simulink model "M2C_IM_CL_V1_NCADMM_Sim"  (R2023a)
settings: Solver=ode4  StartTime=0.0  StopTime=t_sim  FixedStep=tsim  RelTol=1e-3
model workspace (MAT data in the model file):
  global_can_baud_rate = '1000000'
  global_ip_addresses : object (value not decoded)
values from neighbouring files (symbols this model uses):
  A = [1 1 1 0 0 0 ... (first row only)    [M2C_init.m]    (also in MMCC_Sim_Script_BCD_activeset.m = -[1 0 0 1 0 0 1 0 0; 0 1 0 0 1 0 0 1 0; 0 0 1 0 0 1 0 0 1; -; MMCC_Sim_Script_BCD_activeset_LH.m = -[1 0 0 1 0 0 1 0 0; 0 1 0 0 1 0 0 1 0; 0 0 1 0 0 1 0 0 1; -)
  A11 = -(1/tau_sig)*eye(2)    [M2C_init.m]
  A21 = (Lm/tau_r)*eye(2)    [M2C_init.m]
  A_admm = zeros(2*Np, Np)    [M2C_init.m]
  A_cc = [1 0 ... (first row only)    [M2C_init.m]
  b_admm_1 = imax_admm*ones(2*Np,1)    [M2C_init.m]
  b_cc = Vmax_cc*ones(4,1)    [M2C_init.m]
  c_admm = -imax_admm*ones(Np,1)    [M2C_init.m]
  C_obs = [eye(2) zeros(2)]    [M2C_init.m]
  C_sm = 987e-6    (= 0.000987)    [M2C_init.m]
  G_cc = [1 1 ... (first row only)    [M2C_init.m]
  J_imag = [0 -1 ... (first row only)    [M2C_init.m]
  K_obsm = K_obs2'    [M2C_init.m]
  K_obsp = K_obs1'    [M2C_init.m]
  kr = Lm/Lr    (= 0.989061842659)    [M2C_init.m]
  L = 5e-3    (= 0.005)    [M2C_init.m]    (also in MMCC_Sim_Script_BCD_activeset.m = 0.02; MMCC_Sim_Script_BCD_activeset_LH.m = 0.02)
  Lsigmar = 2.6e-3    (= 0.0026)    [M2C_init.m]
  Lsigmas = 2.6e-3    (= 0.0026)    [M2C_init.m]
  N = [1/sqrt(3) 0;-1/(2*sqrt(3)) 1/2;-1/(2*sqrt(3)) -1/2;-1/sqrt(3) 0;1/(2*sqrt(3)) -1/2;1/(2*sqrt(3)) 1/2]    [M2C_init.m]    (also in MMCC_Sim_Script_BCD_activeset.m = null(A,'rational'); MMCC_Sim_Script_BCD_activeset_LH.m = [-0.4430   -0.4780    0.0994    0.0994)
  n = 4    [M2C_init.m]
  p = 2    [M2C_init.m]
  phirN = 1*Vb/ws_nom    [M2C_init.m]
  prmt_ADMM = [n, lambda_z, rho, lambda_e, C_sm, Np, imax_admm]    [M2C_init.m]
  prmt_bkpsi = [ts, Np, lambda_o, imax_admm]    [M2C_init.m]
  prmt_CCMPC = [ts, L, lambda_u, lambda_i, R, e]    [M2C_init.m]
  prmt_OBS = [ts, kr, sigma, Ls, tau_r]    [M2C_init.m]
  R = 0.2    [M2C_init.m]    (also in MMCC_Sim_Script_BCD_activeset.m = 0.001; MMCC_Sim_Script_BCD_activeset_LH.m = 0.001)
  Rr = 1.8    [M2C_init.m]
  Rs = 1.8    [M2C_init.m]
  Rsig = Rs + Rr*kr^2    (= 3.56083799149)    [M2C_init.m]
  SN = PN/FPn    (= 3703.7037037)    [M2C_init.m]
  T = [An ... (first row only)    [M2C_init.m]    (also in MMCC_Sim_Script_BCD_activeset.m = [1   0 ; -1/2  sqrt(3)/2; -1/2  -sqrt(3)/2]; MMCC_Sim_Script_BCD_activeset_LH.m = [1   0 ; -1/2  sqrt(3)/2; -1/2  -sqrt(3)/2])
  t_arranque = t_flux + 5/(dam*wn_flux) + 0.4    [M2C_init.m]
  t_flux = t_maq + 0.1    (= 0.3)    [M2C_init.m]
  t_load = t_arranque    [M2C_init.m]
  Tab0 = (1/3)*[2 -1 -1 ... (first row only)    [M2C_init.m]
  Tabc = [1 0; -.5 sqrt(3)/2; -.5 -sqrt(3)/2]    [M2C_init.m]
  tau_r = Lr/Rr    (= 0.132055555556)    [M2C_init.m]
  TN = PN/(nN*pi/30)    (= 19.7571653493)    [M2C_init.m]
  ts = 1/fs    (= 0.000166666666667)    [M2C_init.m]
  tsim = ts/40    (= 4.16666666667e-06)    [M2C_init.m]
  Vc0 = n*Vc_sm    (= 520)    [M2C_init.m]    (also in MMCC_Sim_Script_BCD_activeset.m = 18000; MMCC_Sim_Script_BCD_activeset_LH.m = 18000)
  Vc_sm = 130    [M2C_init.m]
  Vdc = n*Vc_sm    (= 520)    [M2C_init.m]
undefined symbols (not defined in the file or in its folder): Down, M2C_ADMM_Init_IM_V1, plecs, Up
libraries: spsIGBTDiodeLib x48, spsVoltageMeasurementLib x36, spsSeriesRLCBranchLib x30, spsCurrentMeasurementLib x10, eePwmGenerator x6, rtlab x3, dspstat3 x2, spsControlledVoltageSourceLib x2, spsDCVoltageSourceLib x2, opal_lib x1, dspfdesign x1, spsMeanLib x1
(part 6 of 6)

== matlab function M2C_IM_CL_V1_NCADMM_Sim/SM_MainCPU/Flux obs ==
  settings: updateMethod=DISCRETE  sampleTime=ts
  data: in input; psi_mag output; prmt_OBS parameter; psi_ang output; w_s output; A11 parameter; A21 parameter; C_obs parameter; J_imag parameter; K_obsp parameter; K_obsm parameter
function [psi_mag,psi_ang, w_s] = fcn(in, prmt_OBS, A11, A21, C_obs, J_imag, K_obsp, K_obsm)

persistent x
if isempty(x)
    x = zeros(4,1);
end 

Ts = prmt_OBS(1); kr = prmt_OBS(2); sigma = prmt_OBS(3);
Ls = prmt_OBS(4); tau_psi = prmt_OBS(5);

is_albet = [in(1); in(2)];
w = in(3);

A12 = (kr/(sigma*Ls))*((1/tau_psi)*eye(2) - w*J_imag);
A22 = -((1/tau_psi)*eye(2) - w*J_imag);

A_obs = [A11*0 A12*0;
         A21 A22];
Ad_obs = eye(4) + A_obs*Ts + 0.5*A_obs*A_obs*(Ts^2);

if w < 0
    K_obs = K_obsm;
else
    K_obs = K_obsp;
end

% x_k1 = Ad_obs*x + Bd_obs*vs_albet + K_obs*(is_albet - C_obs*x);
x_k1 = Ad_obs*x + K_obs*(is_albet - C_obs*x);
En = 1;
psi_mag = sqrt(x(3)^2 + x(4)^2);
psi_ang = atan2(x(4), x(3));
if psi_mag == 0 
    w_s = 0;
else
    w_s = (x(3)*(x_k1(4) - x(4))/Ts - x(4)*(x_k1(3) - x(3))/Ts)/(psi_mag^2);
end

x = x_k1;

== matlab function M2C_IM_CL_V1_NCADMM_Sim/SM_MainCPU/Flux Control Proportional Control ==
  settings: updateMethod=DISCRETE  sampleTime=ts
  data: in input; id_ref output; prmt_FC parameter; En input
function id_ref = fcn(in, prmt_FC, En)
% 3 inputs
% 1 output
% 5 parameters

psir = in(1);
psir_ref = in(2);

Kpt = prmt_FC(1)/1.5;
imax = prmt_FC(2);
ts = prmt_FC(3);
Lm = prmt_FC(4);

im_r = psir/Lm;
im_rr = psir_ref/Lm;

im_rr = im_rr*(Kpt + 1)/Kpt;

% nct = 1 - ts*0.5*Kit/Kpt;

% error
persistent a 
if isempty(a)
    a = 0;
end

% % antiwindup signal
persistent u
if isempty(u)
    u = 0;
end


%% PI antiwindup
e1 = (im_rr - im_r);


% a = (nct - 1)*u/Kpt + a*nct;
% u = (e1 - a)*Kpt;


% if u >= imax
%     u = imax;
% elseif u <= -imax
%     u = -imax;
% end

u2 = Kpt*e1;

if u2 >= imax
    u2 = imax;
elseif u2 <= -imax
    u2 = -imax;
end

id_ref = En*u2;

== matlab function M2C_IM_CL_V1_NCADMM_Sim/SM_MainCPU/Output Current Control Proportional Integral Control1 ==
  settings: updateMethod=DISCRETE  sampleTime=ts
  data: id_in input; iq_in input; vd_ref output; vq_ref output; prmt_OCC parameter; w_s input; En input; f input
function [vd_ref, vq_ref] = fcn(id_in, iq_in, prmt_OCC, w_s, En, f)
% 3 inputs
% 1 output
% 5 parameters

id = id_in(1);
id_ref = id_in(2);


iq = iq_in(1);
iq_ref = iq_in(2);

Kct = prmt_OCC(1);
nct = prmt_OCC(2);
vmax = prmt_OCC(3);
% ts = prmt_OCC(4);
L_eq = prmt_OCC(5);

% nct = 1 - ts*0.5*Kit/Kpt;

% error
persistent ad 
if isempty(ad)
    ad = 0;
end

% % antiwindup signal
persistent ud
if isempty(ud)
    ud = 0;
end

% error
persistent aq 
if isempty(aq)
    aq = 0;
end

% % antiwindup signal
persistent uq
if isempty(uq)
    uq = 0;
end

%% PI antiwindup
ed = (id_ref - id);
eq = (iq_ref - iq);

ad = (nct - 1)*ud/Kct + ad*nct;
ud = (ed - ad)*Kct;


aq = (nct - 1)*uq/Kct + aq*nct;
uq = (eq - aq)*Kct;

mag_u = sqrt(ud^2 + uq^2);
ang_u = atan2(uq,ud);

if mag_u >= f*vmax
    mag_u = f*vmax;
elseif mag_u <= -f*vmax
    mag_u = -f*vmax;
end

vd_ref = En*(mag_u*cos(ang_u) - w_s*L_eq*iq*1);
vq_ref = En*(mag_u*sin(ang_u) + w_s*L_eq*id*1);

== matlab function M2C_IM_CL_V1_NCADMM_Sim/SM_MainCPU/Derivada ==
  settings: updateMethod=DISCRETE  sampleTime=ts
  data: x input; dx output; ts parameter
function dx = fcn(x, ts)

persistent x0

if isempty(x0)
    x0 = 0;
end 
dtheta = (x - x0);
dx = 0;

if dtheta > -pi && dtheta < pi 
    dx = dtheta/(ts);
elseif dtheta < -pi
    dx = (dtheta + 2*pi)/(ts);
elseif dtheta > pi
    dx = (dtheta - 2*pi)/(ts);
end

if dx < -200*pi
    dx = -200*pi;
elseif dx > 200*pi
    dx = 200*pi;
end

x0 = x;

== matlab function M2C_IM_CL_V1_NCADMM_Sim/SM_MainCPU/ADMM Horizonte Np/bk & ΔΨ0 1 ==
  settings: updateMethod=DISCRETE  sampleTime=ts
  data: v_dc_ab input; prmt_bkpsi parameter; i_dc_albet input; w_m input; v_o input; Tab0 parameter; A parameter; Tabc parameter; deb output; N parameter; b_k output; i_xyl output; psi0_k output; lambda_o input; En input
function [deb, b_k, i_xyl, psi0_k] = fcn(v_dc_ab, prmt_bkpsi, i_dc_albet, w_m, v_o, Tab0, A, Tabc, N, lambda_o, En)
% 6 inputs
% 6 outputs

% v_dc_abc tensiones en cada nodo vector 5 x 1 [vp vm va vb vc]
% i_dc_albet corriente dc de entrada y componentes alfa y beta de la
% salida vector 3 x 1 [(2/3)*idc -0.5*i_al -0.5*i_bet]
% tensión de modo común escalar

Ts = prmt_bkpsi(1); Np = prmt_bkpsi(2);
% lambda_o = prmt_bkpsi(3); 
imax = prmt_bkpsi(4);
b_k = zeros(Np+1*0,6);
psi0_k = zeros(Np+1*0,6);
i_xyl = zeros(6,Np+1*0);


options = mpcActiveSetOptions;
lb = -imax*ones(6,1);
ub = imax*ones(6,1);
iA0 = false(size([ub;-lb]));
i_z0 = zeros(Np+1,6);

v_albet = [v_dc_ab(3) ; v_dc_ab(4)];
i_albet = [i_dc_albet(1) ; i_dc_albet(2)];
idcl = i_dc_albet(3);
vdcl = [v_dc_ab(1) ; v_dc_ab(2)];

magv_o = v_o(1);
angv_o = v_o(2);
wo = 200*2*pi;
wb = 50*2*pi;

for l = 0:Np-1+1*0
    wt = (l)*Ts*w_m;
    wot = (l)*Ts*wo;
    iabl = [cos(wt) -sin(wt);
           sin(wt) cos(wt)]*i_albet;
    vabl = [cos(wt) -sin(wt);
           sin(wt) cos(wt)]*[v_albet(1) ; v_albet(2)];

    % Transformación
    vabcl = Tabc*vabl;
    iabcl = Tabc*iabl;
    v_l = [vdcl ; vabcl];
    v_xyl = A'*v_l;  % [vpa vpb vpc vma vmb vmc] 6 x 1
    ipa = 0.333*idcl - 0.5*iabcl(1);
    ipb = 0.333*idcl - 0.5*iabcl(2);
    ipc = 0.333*idcl - 0.5*iabcl(3);

    ima = -0.333*idcl - 0.5*iabcl(1);
    imb = -0.333*idcl - 0.5*iabcl(2);
    imc = -0.333*idcl - 0.5*iabcl(3);
    
    i_xyl(:,l+1) = [ipa ; ipb ; ipc ; ima ; imb ; imc];

    v_o = magv_o*(cos(angv_o)*sin(wot) + sin(angv_o)*cos(wot));
    if v_o > 0.7*500*0.5*(1 - abs(wt)/wb)
        v_o = 0.7*500*0.5*(1 - abs(wt)/wb);
    elseif v_o < -0.7*500*0.5*(1 - abs(wt)/wb)
        v_o = -0.7*500*0.5*(1 - abs(wt)/wb);
    end
    if v_o > 0.7*500*0.5
        v_o = 0.7*500*0.5;
    elseif v_o < -0.7*500*0.5
        v_o = -0.7*500*0.5;
    end

    aux = Ts*(v_xyl + v_o*ones(6,1));

    % vxy = A'*vxypred(k,:);
%     D = diag(v_xyl);
%     Do = diag(v_o*ones(6,1));
%     H = 2*((Ts^2)*(N'*(D + Do)^2)*N + lambda_o*N'*N);
%     u = Ts*(D + Do)*i_xyl(:,l+1);
%     f = 2*Ts*N'*(D + Do)*u;
% 
%     [Z, ~] = mpcActiveSetSolver(H,f,[N;-N],[ub;-lb],zeros(0,length(f)),zeros(0,1),iA0,options);
%     i_z0(l+1,:) = N*Z;

    b_k(l+1,:) = aux';
    psi0_k(l+1,:) = (aux.*i_xyl(:,l+1))';
end
deb = iabcl(2);

== matlab function M2C_IM_CL_V1_NCADMM_Sim/SM_MainCPU/Speed Control Proportional Integral Control ==
  settings: updateMethod=DISCRETE  sampleTime=6*ts
  data: in input; iq_ref output; prmt_SC parameter; En input
function iq_ref = fcn(in, prmt_SC, En)
% 3 inputs
% 1 output
% 5 parameters

w = in(1);
w_ref = in(2);

Kpt = prmt_SC(1);
nct = prmt_SC(2);
imax = prmt_SC(3);
% Adc = prmt_SC(4);
ts = prmt_SC(4);

% nct = 1 - ts*0.5*Kit/Kpt;

% error
persistent a 
if isempty(a)
    a = 0;
end

% % antiwindup signal
persistent u
if isempty(u)
    u = 0;
end


%% PI antiwindup
e1 = (w_ref - w);

a = (nct - 1)*u/Kpt + a*nct;
u = (e1 - a)*Kpt;

if u >= imax
    u = imax;
elseif u <= -imax
    u = -imax;
end


iq_ref = En*u;

== matlab function M2C_IM_CL_V1_NCADMM_Sim/SM_MainCPU/Flux obs1 ==
  settings: updateMethod=DISCRETE  sampleTime=ts
  data: in input; psi_mag output; prmt_EST parameter; w_s output
function [psi_mag, w_s] = fcn(in, prmt_EST)

persistent psir0
if isempty(psir0)
    psir0 = 0;
end 

Ts = prmt_EST(1); tau_r = prmt_EST(2); Lm = prmt_EST(3);

is_dq = [in(1); in(2)];
w = in(3);

psi_mag = (Lm*is_dq(1) + (tau_r/Ts)*psir0)/(tau_r/Ts + 1);

if psi_mag == 0 
    w_r = 0;
else
    w_r = Lm*is_dq(2)/(tau_r*psi_mag);
end

w_s = w_r + w;

psir0 = psi_mag;

== matlab function M2C_IM_CL_V1_NCADMM_Sim/SM_MainCPU/n_ref ==
  settings: updateMethod=DISCRETE  sampleTime=ts
  data: time input; n_ref output; En input; fw input; n_max input; n_min input; n_sl input; t_max input
function n_ref = fcn(time, En, fw, n_max, n_min, n_sl, t_max)

persistent x
if isempty(x)
    x = 0;
end 
persistent x1
if isempty(x1)
    x1 = 0;
end 

persistent n0
if isempty(n0)
    n0 = 0;
end 
persistent n01
if isempty(n01)
    n01 = 0;
end 

persistent t0
if isempty(t0)
    t0 = 0;
end 
persistent t1
if isempty(t1)
    t1 = 0;
end 
% n_max = 750;
if En == 1 && x == 0
    t0 = time;
end

if En == 1 && x1 == 0
    t1 = time;
end
if En == 1
    if fw == 1
        dt = time - t0;
        n_ref = n0 + (n_sl/t_max)*dt;
        x = 1;
        x1 = 0;
        n01 = n_max;
    else
        dt = time - t1;
        n_ref = n01 - (n_sl/t_max)*dt;
        x1 = 1;
        x = 0;
        n0 = n_min;
    end
else
    n_ref = 0;
end
if n_ref < n_min
    n_ref = n_min;
elseif n_ref > n_max
    n_ref = n_max;
end

== matlab function M2C_IM_CL_V1_NCADMM_Sim/SM_MainCPU/BCD CEC-MPC ==
  data: Vck input; Vcp input; ixy input; Vxab input; Vypn input; wx input; wy input; von output; t input; lambdav input; izo output; lambdaz input
function [von,izo]  = fcn(Vck,Vcp,ixy,Vxab,Vypn,wx,wy,t,lambdav,lambdaz)
% transformada doble alpha beta 0
%C=4.7e-3;
%C=20e-3;
C=987e-6;
%Tp=1/50/4;%Tiempo de horizonte de prediccion. 1 ciclo de la oscilación de baja frecuencia
%Tp=0.0006;
%Tp=0.001;
Ts=1/6000;%Tiempo de muestreo
%Np=Tp/Ts;%Puntos del horizonte de prediccion.
Np=1;
%DV=DV0;
%DI=DI0;
lM=15;
gap=0.01;
DV=zeros(6*Np,6*Np);
DI=zeros(6*Np,Np);
Dn=zeros(6*Np,6*Np);
A=[1 1 1 0 0 0;0 0 0 1 1 1; -1 0 0 -1 0 0;0 -1 0 0 -1 0; 0 0 -1 0 0 -1];
At=repmat({A},1,Np);
At=blkdiag(At{:});
%lambdav=5e-3; %lazo de corriente lento
%lambdaz=5e-1;
Ilb=-10*ones(6*Np,1);
Iub=10*ones(6*Np,1);
%lambdav=6e-3; %lazo de corriente rapido
%lambdaz=1e-1;
Y=zeros(6,Np); 
von=0;
N=[1/sqrt(3) 0;-1/(2*sqrt(3)) 1/2;-1/(2*sqrt(3)) -1/2;-1/sqrt(3) 0;1/(2*sqrt(3)) -1/2;1/(2*sqrt(3)) 1/2];
N1=repmat({N(:,1)},1,Np);
N1=blkdiag(N1{:});
N2=repmat({N(:,2)},1,Np);
N2=blkdiag(N2{:});
iz1p=zeros(Np,1);
iz2p=zeros(Np,1);
fval0=0;
efr=1;
l=0;
final_ub=zeros(6,1);
final_lb=zeros(6,1);
ex=int32(0);
%Future Currents
X=ixy;
ixypred=zeros(6,Np);
tp=linspace(0,Np*Ts,Np);
iab0xpred=(X(1)+j*X(2))*exp(j*wx*tp);
iab0ypred=(X(3)+j*X(4))*exp(j*wy*tp);
%if vonM>260
    vonmax=260;
%else
%    vonmax=vonM;
%end
%if vonm<-260
    vonmin=-260;
%else
%    vonmin=vonm;
%end
persistent izp
if isempty(izp)
    izp=zeros(6,Np);
end
persistent iA0v
if isempty(iA0v)
    iA0v=false(size([ones(Np,1);ones(Np,1)]));
end
persistent iA01
if isempty(iA01)
    iA01=false(size([ones(6*Np,1);ones(6*Np,1)]));
end
persistent iA02
if isempty(iA02)
    iA02=false(size([ones(6*Np,1);ones(6*Np,1)]));
end
for k=1:Np
    Xa0=-real(iab0xpred(k)); Xb0=-imag(iab0xpred(k)); 
    X0a=real(iab0ypred(k)); X0b=imag(iab0ypred(k));
    P=pinv([1 1 1 0 0 0;0 0 0 1 1 1; -1 0 0 -1 0 0;0 -1 0 0 -1 0; 0 0 -1 0 0 -1]);
    Tabc=[1 0;-1/2 sqrt(3)/2;-1/2 -sqrt(3)/2];
    ixypred(:,k)=P*[X0a;X0b;Tabc*[Xa0;Xb0]];
    %Y(7,k)=YAc; Y(8,k)=YBc; Y(9,k)=YCc;
end
    %Future Voltages
    vxypred=zeros(5,Np);
    vab0xpred=(Vxab(1)+j*Vxab(2))*exp(j*wx*tp);
    T=[ 1   0 ; -1/2  sqrt(3)/2; -1/2  -sqrt(3)/2]; %Trans Alpha-Beta to abc
    for k=1:Np
        vabc=T*[real(vab0xpred(k));imag(vab0xpred(k))];
        vxypred(1,k)=vabc(1); vxypred(2,k)=vabc(2); vxypred(3,k)=vabc(3);
        vxypred(4,k)=Vypn(1); vxypred(5,k)=Vypn(2);
        vxy=A'*vxypred(:,k);
        DV((6*k-5):6*Np,(6*k-5):6*k)=repmat(diag(vxy),Np+1-k,1);
    end

l=0;
rel=[1,1,1];
if t>0.1
    iA1=false(size([Iub;-Ilb]));
    iA2=false(size([Iub;-Ilb]));
    lmax=lM;
    Jv0=1000000;
    Jv1=0;
    Je10=1000000;
    Je11=0;
    Je20=1000000;
    Je21=0;
    relv=abs(Jv1-Jv0)/abs(Jv0);
    rele1=abs(Je11-Je10)/abs(Je10);
    rele2=abs(Je21-Je20)/abs(Je20);
    rel=[relv,rele1,rele2];
    while any(rel>gap)
        l=l+1;
        %if t>0.35
        %    izp(:,1)=iz;
        %end
    
        for k=1:Np
            DI((6*k-5):6*Np,k)=repmat(ixypred(:,k)+izp(:,k),Np+1-k,1);
        end
        Eck=(C*Vck.*Vck/4)/2;
        Ecref=C*500^2*ones(6,1)/2;
        Ecprom=(C/4)*Vcp^2*ones(6,1)/2;
        y=repmat(Eck,Np,1)+Ts*DV*reshape(ixypred+izp,[6*Np,1])-repmat(Ecprom,Np,1);
        H=2*((Ts)^2*transpose(DI)*DI+lambdav*eye(Np));
        f=2*Ts*transpose(DI)*y;
        %x0 = zeros(Np,1);
        %options = optimoptions('quadprog','Algorithm','active-set');
        %ws = optimwarmstart(x0,options);
        lb=vonmin*ones(Np,1);
        ub=vonmax*ones(Np,1);
        %Z=quadprog(H,f,[],[],[],[],lb,ub,ws);
        options = mpcActiveSetOptions;
        options.MaxIterations = 10;
        options.ConstraintTolerance = 1.0e-3;
        [ZX,exitflag,iA0,mu]=mpcActiveSetSolver(H,f,[eye(Np);-eye(Np)],[ub;-lb],zeros(0,length(f)),zeros(0,1),iA0v,options); 
        Jv1=0.5*ZX'*H*ZX+f'*ZX;
        relv=abs(Jv1-Jv0)/abs(Jv0);
        Jv0=Jv1;
        iA0v=iA0;
        von=ZX(1);
        vonpred=ZX;    
        if von>vonmax
            von=vonmax;
        elseif von<vonmin
            von=vonmin;
        end
        Y=zeros(6,Np);
        for k=1:Np
           Dn((6*k-5):6*Np,(6*k-5):6*k)=repmat(vonpred(k)*eye(6),Np+1-k,1);
        end
        Dt=Dn+DV;
        H=2*((Ts)^2*transpose(Dt*N1)*(Dt*N1)+lambdaz*(N1')*N1); 
        dz=repmat(Eck,Np,1)-repmat(Ecprom,Np,1)+Ts*Dt*reshape(ixypred,[6*Np,1])+Ts*Dt*N2*iz2p;
        f=2*Ts*transpose(Dt*N1)*dz+2*lambdaz*(iz2p'*N2'*N1)';
        %beq = repmat([0 0 0 0 0],[Np,1]);
        %options = optimoptions('quadprog','Algorithm','active-set');
        %ws = optimwarmstart(iz1p,options);
        %Zz=quadprog(H,f,[],[],[],[],-1500*ones(Np,1),1500*ones(Np,1),ws);
        ub=Iub-reshape(ixypred,[6*Np,1])-N2*iz2p;
        lb=Ilb-reshape(ixypred,[6*Np,1])-N2*iz2p;
        [Z1,exitflag,iA1,lambda]=mpcActiveSetSolver(H,f,[N1;-N1],[ub;-lb],zeros(0,length(f)),zeros(0,1),iA01,options);  
        Je11=0.5*Z1'*H*Z1+f'*Z1;
        rele1=abs(Je11-Je10)/abs(Je10);
        Je10=Je11;
        iA01=iA1;
        %options = mpcInteriorPointOptions;
        %options.MaxIterations = 5;
        %options.ConstraintTolerance = 1.0e-3;
        %[Z1,exitflag]=mpcInteriorPointSolver(H,f,[N1;-N1],[ub;-lb],zeros(0,length(f)),zeros(0,1),iz1p,options);         
        iz1p=Z1;
    
        H=2*((Ts)^2*transpose(Dt*N2)*(Dt*N2)+lambdaz*(N2')*N2); 
        dz=repmat(Eck,Np,1)-repmat(Ecprom,Np,1)+Ts*Dt*reshape(ixypred,[6*Np,1])+Ts*Dt*N1*iz1p;
        f=2*Ts*transpose(Dt*N2)*dz+2*lambdaz*(iz1p'*N1'*N2)';
        ub=Iub-reshape(ixypred,[6*Np,1])-N1*iz1p;
        lb=Ilb-reshape(ixypred,[6*Np,1])-N1*iz1p;
        [Z2,exitflag,iA2,lambda]=mpcActiveSetSolver(H,f,[N2;-N2],[ub;-lb],zeros(0,length(f)),zeros(0,1),iA02,options);    
        Je21=0.5*Z2'*H*Z2+f'*Z2;
        rele2=abs(Je21-Je20)/abs(Je20);
        Je20=Je21;
        iA02=iA2;
        %[Z2,exitflag]=mpcInteriorPointSolver(H,f,[N2;-N2],[ub;-lb],zeros(0,length(f)),zeros(0,1),iz2p,options);      
        iz2p=Z2;
        %z21=iz2p(1);
        %z22=Z2(1);
        %fval1=0.5*Z2'*H*Z2+f'*Z2;
        %efr=abs((fval1-fval0)/fval1);
        %fval0=fval1;
        izpalt=reshape(N1*iz1p+N2*iz2p,[6,Np]);
        Y=izpalt;
        izp=Y;
        %final_ub_out=Iub-double(reshape(ixypred,[6*Np,1]))-N1*iz1p-N2*iz2p;
        %final_lb_out=Ilb-double(reshape(ixypred,[6*Np,1]))-N1*iz1p-N2*iz2p;
        %final_ub=final_ub_out(1:6);
        %final_lb=final_lb_out(1:6);
        %ex=exitflag;
        rel=[relv,rele1,rele2];
        if l>lmax
            break
        end
          
    end    
    %options = mpcActiveSetOptions;
    %[Zz,exitflag]=mpcActiveSetSolver(H,f,[N1;-N1],[ub;lb],zeros(0,length(f)),zeros(0,1),iA0,options);
else
end
Iub=reshape(Iub,[6,Np]);
Ilb=reshape(Ilb,[6,Np]);
if any(Y>Iub)
    Y=min(Y,Iub);
elseif any(Y<Ilb)
    Y=max(Y,Ilb);
end
izpred1=Y;  
izo=izpred1(:,1);

== matlab function M2C_IM_CL_V1_NCADMM_Sim/SM_MainCPU/From abc to αβ0^2.1 ==
  data: X input; Y output
function Y = fcn(X)
% transformada doble alpha beta 0
XAa=X(1); XBa=X(2); XCa=X(3);
XAb=X(4); XBb=X(5); XCb=X(6);
XAc=0; XBc=0; XCc=0;

Yaa= 0.666667*XAa - 0.333333*XAb - 0.333333*XAc - 0.333333*XBa + 0.166667*XBb + 0.166667*XBc - 0.333333*XCa + 0.166667*XCb + 0.166667*XCc;
Yba= 0.57735*XBa - 0.288675*XBb - 0.288675*XBc - 0.57735*XCa + 0.288675*XCb + 0.288675*XCc;
Y0a= 0.471405*XAa - 0.235702*XAb - 0.235702*XAc + 0.471405*XBa -  0.235702*XBb - 0.235702*XBc + 0.471405*XCa - 0.235702*XCb -  0.235702*XCc;

Yab= 0.57735*XAb - 0.57735*XAc - 0.288675*XBb + 0.288675*XBc - 0.288675*XCb + 0.288675*XCc;
Ybb= 0.5*XBb - 0.5*XBc - 0.5*XCb + 0.5*XCc;
Y0b= 0.408248*XAb - 0.408248*XAc + 0.408248*XBb - 0.408248*XBc + 0.408248*XCb - 0.408248*XCc;

Ya0= 0.471405*XAa + 0.471405*XAb + 0.471405*XAc - 0.235702*XBa - 0.235702*XBb - 0.235702*XBc - 0.235702*XCa - 0.235702*XCb - 0.235702*XCc;
Yb0= 0.408248*XBa + 0.408248*XBb + 0.408248*XBc - 0.408248*XCa - 0.408248*XCb - 0.408248*XCc;
Y00= 0.333333*XAa + 0.333333*XAb + 0.333333*XAc + 0.333333*XBa + 0.333333*XBb + 0.333333*XBc + 0.333333*XCa + 0.333333*XCb + 0.333333*XCc;

Y=zeros(9,1);
Y(1)=Yaa; Y(2)=Yba; Y(3)=Y0a;
Y(4)=Yab; Y(5)=Ybb; Y(6)=Y0b;
Y(7)=sqrt(2)*Ya0; Y(8)=sqrt(2)*Yb0; Y(9)=Y00;

== matlab function M2C_IM_CL_V1_NCADMM_Sim/SM_MainCPU/dq --> ab1 ==
  settings: updateMethod=DISCRETE  sampleTime=ts
  data: dq input; ab output; Theta_s input
function ab = fcn(dq, Theta_s)

Tab = [cos(Theta_s) -sin(Theta_s);
      sin(Theta_s) cos(Theta_s)];
ab = Tab*dq;

== matlab function M2C_IM_CL_V1_NCADMM_Sim/SM_MainCPU/LCB1/Greedy3 ==
  settings: updateMethod=DISCRETE  sampleTime=ts
  data: Vc_xy input; i_xy input; m_xy output; prmt_LCB parameter; Vcr_xy input; EN input; Op_all input; EN_TEB input
function m_xy  = fcn(Vc_xy, i_xy, prmt_LCB, Vcr_xy, EN, Op_all, EN_TEB)

%% Local Balance P controller
n = prmt_LCB(1) ; Vc_prom = prmt_LCB(2); Kc = prmt_LCB(3);

m_xyh = zeros(4,2);
% m_xyl = zeros(4,1);

Vc1 = Vc_xy(1) ; Vc2 = Vc_xy(2); Vc3 = Vc_xy(3); Vc4 = Vc_xy(4);

% d1 = (Vc_prom - Vc1);
% d2 = (Vc_prom - Vc2);
% d3 = (Vc_prom - Vc3);
% d4 = (Vc_prom - Vc4);

d = [Vc1 1; Vc2 2; Vc3 3; Vc4 4];
st_two_w = zeros(2,2);
st_two_l = zeros(2,2);

st_three = zeros(2,2);

% Stage 1 
if Vc1 > Vc2
    st_two_w(1,:) = d(1,:);
    st_two_l(1,:) = d(2,:);
else
    st_two_w(1,:) = d(2,:);
    st_two_l(1,:) = d(1,:);
end
if Vc3 > Vc4
    st_two_w(2,:) = d(3,:);
    st_two_l(2,:) = d(4,:);
else
    st_two_w(2,:) = d(4,:);
    st_two_l(2,:) = d(3,:);
end

% Stage 2
if st_two_w(1,1) > st_two_w(2,1)
    m_xyh(1,:) = st_two_w(1,:);
    st_three(1,:) = st_two_w(2,:);
else
    m_xyh(1,:) = st_two_w(2,:);
    st_three(1,:) = st_two_w(1,:);
end
if st_two_l(1,1) < st_two_l(2,1)
    m_xyh(4,:) = st_two_l(1,:);
    st_three(2,:) = st_two_l(2,:);
else
    m_xyh(4,:) = st_two_l(2,:);
    st_three(2,:) = st_two_l(1,:);
end

%Stage 3
if st_three(1,1) > st_three(2,1)
    m_xyh(2,:) = st_three(1,:);
    m_xyh(3,:) = st_three(2,:);
else
    m_xyh(2,:) = st_three(2,:);
    m_xyh(3,:) = st_three(1,:);
end

if sign(i_xy) > 0
    m_xyh = flip(m_xyh);
end

u_xy = m_xyh(:,1); % Orden de tensiones
n_xy = m_xyh(:,2); % Submodulo al que pertenecen

m_xy = zeros(4,1);
u_sigma = 0;

for i = 1:4
    l = n_xy(i);
    if u_sigma + u_xy(i) <= Vcr_xy
        m_xy(l) = 1;
        u_sigma = u_sigma + u_xy(i);
    else
        m_xy(l) = (Vcr_xy - u_sigma)/u_xy(i);
        if m_xy(l) < 0
            m_xy(l) = 0;
        end
%         if m_xy(l) > 1
%             m_xy(l) = 1;
%         end
        break
    end
end

% m_xy = EN*m_xy;


if Op_all == 1 && EN_TEB == 0
    m_xy = ones(4,1);
else
    m_xy = EN*m_xy;
end






% % Sort h
% for i = 1:4
%     for j = 1:4
%     if i ~= j
%         if d(i) > d(j)
%             m_xyh(i) = m_xyh(i) + 1;
%         end
%     end
%     end
% end
% 
% % Sort l
% for i = 1:4
%     for j = 1:4
%     if i ~= j
%         if d(i) < d(j)
%             m_xyl(i) = m_xyl(i) + 1;
%         end
%     end
%     end
% end
% 
% if sign(i_xy) >= 0
%     m_xy = m_xyh;
% else
%     m_xy = m_xyl;
% end



% for i = 1:4
%     m_xy(i) = Vcrp(i) + d(i);
% end

== matlab function M2C_IM_CL_V1_NCADMM_Sim/SM_MainCPU/LCB1/Greedy4 ==
  settings: updateMethod=DISCRETE  sampleTime=ts
  data: Vc_xy input; i_xy input; m_xy output; prmt_LCB parameter; Vcr_xy input; EN input; Op_all input; EN_TEB input
function m_xy  = fcn(Vc_xy, i_xy, prmt_LCB, Vcr_xy, EN, Op_all, EN_TEB)

%% Local Balance P controller
n = prmt_LCB(1) ; Vc_prom = prmt_LCB(2); Kc = prmt_LCB(3);

m_xyh = zeros(4,2);
% m_xyl = zeros(4,1);

Vc1 = Vc_xy(1) ; Vc2 = Vc_xy(2); Vc3 = Vc_xy(3); Vc4 = Vc_xy(4);

% d1 = (Vc_prom - Vc1);
% d2 = (Vc_prom - Vc2);
% d3 = (Vc_prom - Vc3);
% d4 = (Vc_prom - Vc4);

d = [Vc1 1; Vc2 2; Vc3 3; Vc4 4];
st_two_w = zeros(2,2);
st_two_l = zeros(2,2);

st_three = zeros(2,2);

% Stage 1 
if Vc1 > Vc2
    st_two_w(1,:) = d(1,:);
    st_two_l(1,:) = d(2,:);
else
    st_two_w(1,:) = d(2,:);
    st_two_l(1,:) = d(1,:);
end
if Vc3 > Vc4
    st_two_w(2,:) = d(3,:);
    st_two_l(2,:) = d(4,:);
else
    st_two_w(2,:) = d(4,:);
    st_two_l(2,:) = d(3,:);
end

% Stage 2
if st_two_w(1,1) > st_two_w(2,1)
    m_xyh(1,:) = st_two_w(1,:);
    st_three(1,:) = st_two_w(2,:);
else
    m_xyh(1,:) = st_two_w(2,:);
    st_three(1,:) = st_two_w(1,:);
end
if st_two_l(1,1) < st_two_l(2,1)
    m_xyh(4,:) = st_two_l(1,:);
    st_three(2,:) = st_two_l(2,:);
else
    m_xyh(4,:) = st_two_l(2,:);
    st_three(2,:) = st_two_l(1,:);
end

%Stage 3
if st_three(1,1) > st_three(2,1)
    m_xyh(2,:) = st_three(1,:);
    m_xyh(3,:) = st_three(2,:);
else
    m_xyh(2,:) = st_three(2,:);
    m_xyh(3,:) = st_three(1,:);
end

if sign(i_xy) > 0
    m_xyh = flip(m_xyh);
end

u_xy = m_xyh(:,1); % Orden de tensiones
n_xy = m_xyh(:,2); % Submodulo al que pertenecen

m_xy = zeros(4,1);
u_sigma = 0;

for i = 1:4
    l = n_xy(i);
    if u_sigma + u_xy(i) <= Vcr_xy
        m_xy(l) = 1;
        u_sigma = u_sigma + u_xy(i);
    else
        m_xy(l) = (Vcr_xy - u_sigma)/u_xy(i);
        if m_xy(l) < 0
            m_xy(l) = 0;
        end
%         if m_xy(l) > 1
%             m_xy(l) = 1;
%         end
        break
    end
end

% m_xy = EN*m_xy;


if Op_all == 1 && EN_TEB == 0
    m_xy = ones(4,1);
else
    m_xy = EN*m_xy;
end






% % Sort h
% for i = 1:4
%     for j = 1:4
%     if i ~= j
%         if d(i) > d(j)
%             m_xyh(i) = m_xyh(i) + 1;
%         end
%     end
%     end
% end
% 
% % Sort l
% for i = 1:4
%     for j = 1:4
%     if i ~= j
%         if d(i) < d(j)
%             m_xyl(i) = m_xyl(i) + 1;
%         end
%     end
%     end
% end
% 
% if sign(i_xy) >= 0
%     m_xy = m_xyh;
% else
%     m_xy = m_xyl;
% end



% for i = 1:4
%     m_xy(i) = Vcrp(i) + d(i);
% end

== matlab function M2C_IM_CL_V1_NCADMM_Sim/SM_MainCPU/LCB1/Greedy5 ==
  settings: updateMethod=DISCRETE  sampleTime=ts
  data: Vc_xy input; i_xy input; m_xy output; prmt_LCB parameter; Vcr_xy input; EN input; Op_all input; EN_TEB input
function m_xy  = fcn(Vc_xy, i_xy, prmt_LCB, Vcr_xy, EN, Op_all, EN_TEB)

%% Local Balance P controller
n = prmt_LCB(1) ; Vc_prom = prmt_LCB(2); Kc = prmt_LCB(3);

m_xyh = zeros(4,2);
% m_xyl = zeros(4,1);

Vc1 = Vc_xy(1) ; Vc2 = Vc_xy(2); Vc3 = Vc_xy(3); Vc4 = Vc_xy(4);

% d1 = (Vc_prom - Vc1);
% d2 = (Vc_prom - Vc2);
% d3 = (Vc_prom - Vc3);
% d4 = (Vc_prom - Vc4);

d = [Vc1 1; Vc2 2; Vc3 3; Vc4 4];
st_two_w = zeros(2,2);
st_two_l = zeros(2,2);

st_three = zeros(2,2);

% Stage 1 
if Vc1 > Vc2
    st_two_w(1,:) = d(1,:);
    st_two_l(1,:) = d(2,:);
else
    st_two_w(1,:) = d(2,:);
    st_two_l(1,:) = d(1,:);
end
if Vc3 > Vc4
    st_two_w(2,:) = d(3,:);
    st_two_l(2,:) = d(4,:);
else
    st_two_w(2,:) = d(4,:);
    st_two_l(2,:) = d(3,:);
end

% Stage 2
if st_two_w(1,1) > st_two_w(2,1)
    m_xyh(1,:) = st_two_w(1,:);
    st_three(1,:) = st_two_w(2,:);
else
    m_xyh(1,:) = st_two_w(2,:);
    st_three(1,:) = st_two_w(1,:);
end
if st_two_l(1,1) < st_two_l(2,1)
    m_xyh(4,:) = st_two_l(1,:);
    st_three(2,:) = st_two_l(2,:);
else
    m_xyh(4,:) = st_two_l(2,:);
    st_three(2,:) = st_two_l(1,:);
end

%Stage 3
if st_three(1,1) > st_three(2,1)
    m_xyh(2,:) = st_three(1,:);
    m_xyh(3,:) = st_three(2,:);
else
    m_xyh(2,:) = st_three(2,:);
    m_xyh(3,:) = st_three(1,:);
end

if sign(i_xy) > 0
    m_xyh = flip(m_xyh);
end

u_xy = m_xyh(:,1); % Orden de tensiones
n_xy = m_xyh(:,2); % Submodulo al que pertenecen

m_xy = zeros(4,1);
u_sigma = 0;

for i = 1:4
    l = n_xy(i);
    if u_sigma + u_xy(i) <= Vcr_xy
        m_xy(l) = 1;
        u_sigma = u_sigma + u_xy(i);
    else
        m_xy(l) = (Vcr_xy - u_sigma)/u_xy(i);
        if m_xy(l) < 0
            m_xy(l) = 0;
        end
%         if m_xy(l) > 1
%             m_xy(l) = 1;
%         end
        break
    end
end

% m_xy = EN*m_xy;


if Op_all == 1 && EN_TEB == 0
    m_xy = ones(4,1);
else
    m_xy = EN*m_xy;
end






% % Sort h
% for i = 1:4
%     for j = 1:4
%     if i ~= j
%         if d(i) > d(j)
%             m_xyh(i) = m_xyh(i) + 1;
%         end
%     end
%     end
% end
% 
% % Sort l
% for i = 1:4
%     for j = 1:4
%     if i ~= j
%         if d(i) < d(j)
%             m_xyl(i) = m_xyl(i) + 1;
%         end
%     end
%     end
% end
% 
% if sign(i_xy) >= 0
%     m_xy = m_xyh;
% else
%     m_xy = m_xyl;
% end



% for i = 1:4
%     m_xy(i) = Vcrp(i) + d(i);
% end

== matlab function M2C_IM_CL_V1_NCADMM_Sim/SM_MainCPU/TEB Control Proportional Integral Control ==
  settings: updateMethod=DISCRETE  sampleTime=ts
  data: in input; i_dc output; prmt_TEB parameter; deb output
function [i_dc,deb] = fcn(in, prmt_TEB)
% 3 inputs
% 1 output
% 5 parameters



imax = prmt_TEB(3);
ts = prmt_TEB(7);
wn_teb = prmt_TEB(8);
dam = prmt_TEB(9);
e = prmt_TEB(10);


% Vsc_0 = in(1);
En_total = in(1);
Vdc_ref = in(2);
Pff = in(3);
Vdc = in(4);
En = in(5);


Vsc_0 = En_total;


K_teb = Vdc;

d0_teb = 1; 
n0_teb = ts*K_teb;

aux_teb = -dam*wn_teb*ts;
a1_teb = -2*e^(aux_teb)*cos(wn_teb*ts*sqrt(1-dam^2));
a2_teb = e^(-2*dam*wn_teb*ts);

Kct = (a1_teb + d0_teb + 1)/n0_teb;
nct = (d0_teb - a2_teb)/(a1_teb + d0_teb + 1);


% error
persistent a 
if isempty(a)
    a = 0;
end

% % antiwindup signal
persistent u
if isempty(u)
    u = 0;
end


%% PI antiwindup
e1 = (Vdc_ref - Vsc_0);

a = (nct - 1)*u/Kct + a*nct;
u = (e1 - a)*Kct;


if u >= imax
    u = imax;
elseif u <= -imax
    u = -imax;
end

deb = u;
i_dc = En*(u - 0*Pff/(Vdc));

== matlab function M2C_IM_CL_V1_NCADMM_Sim/SM_MainCPU/I_xy ---> i_x i_y i_xy ==
  data: i_xy_measure input; i_x output; i_y output; i_xy output; A parameter
function [i_x,i_y, i_xy] = fcn(i_xy_measure, A)

i_ap = i_xy_measure(1); i_bp = i_xy_measure(2); i_cp = i_xy_measure(3);
i_an = i_xy_measure(4); i_bn = i_xy_measure(5); i_cn = i_xy_measure(6);

i_xy = [-i_ap; -i_bp; -i_cp; -i_an; -i_bn; -i_cn];

i = A*i_xy;

i_x = i(3:5);
i_y = i(1);

== matlab function M2C_IM_CL_V1_NCADMM_Sim/SM_MainCPU/Vc_kxy --> Vc_xy ==
  settings: updateMethod=DISCRETE  sampleTime=ts
  data: Vc_ap input; Vc_xy output; Vc_bp input; Vc_cp input; Vc_an input; Vc_bn input; Vc_cn input; Ec_xy output; T parameter; E_p output
function [Vc_xy, Ec_xy, E_p] = fcn(Vc_ap, Vc_bp, Vc_cp, Vc_an, Vc_bn, Vc_cn, T)

Vc_xy = zeros(6,1);
Ec_xy = zeros(6,1);

Vc_xy(1) = sum(Vc_ap);
Vc_xy(2) = sum(Vc_bp);
Vc_xy(3) = sum(Vc_cp);
Vc_xy(4) = sum(Vc_an);
Vc_xy(5) = sum(Vc_bn);
Vc_xy(6) = sum(Vc_cn);

Ec_xy(1) = Vc_ap(1)^2 + Vc_ap(2)^2 + Vc_ap(3)^2 + Vc_ap(4)^2;
Ec_xy(2) = Vc_bp(1)^2 + Vc_bp(2)^2 + Vc_bp(3)^2 + Vc_bp(4)^2;
Ec_xy(3) = Vc_cp(1)^2 + Vc_cp(2)^2 + Vc_cp(3)^2 + Vc_cp(4)^2;
Ec_xy(4) = Vc_an(1)^2 + Vc_an(2)^2 + Vc_an(3)^2 + Vc_an(4)^2;
Ec_xy(5) = Vc_bn(1)^2 + Vc_bn(2)^2 + Vc_bn(3)^2 + Vc_bn(4)^2;
Ec_xy(6) = Vc_cn(1)^2 + Vc_cn(2)^2 + Vc_cn(3)^2 + Vc_cn(4)^2;

E_t = 0.5*966e-6*T*Ec_xy;
E_p = E_t(2);

== matlab function M2C_IM_CL_V1_NCADMM_Sim/SM_MainCPU/abc --> dq ==
  settings: updateMethod=DISCRETE  sampleTime=ts
  data: abc input; dq output; Theta_s input
function dq = fcn(abc, Theta_s)

Tdq = 0.6667*[cos(Theta_s) -sin(Theta_s);
              cos(Theta_s - 0.6667*pi) -sin(Theta_s - 0.6667*pi);
              cos(Theta_s + 0.6667*pi) -sin(Theta_s + 0.6667*pi)];
dq = Tdq'*abc;
